simulink model "BE_EGAL_02"  (R2024b)
settings: Solver=ode45  StartTime=0.0  StopTime=Tfinal  RelTol=1e-3  EnableMultiTasking=on
values from neighbouring files (symbols this model uses):
  Constellation = exp(1i*pi*(1+2*kc)/4)    [init_ISI.m]
undefined symbols (not defined in the file or in its folder): dfilt, Limite, Tfinal
libraries: dspobslib x2, commdigbbndam3 x2, commchan3 x1, commsink2 x1, dspstat3 x1, commrandsrc3 x1
settings Model: Creator=Epsilon_2  LastModifiedBy=paulj
settings SolverCC: AlgebraicLoopSolver=TrustRegion
settings DataIOCC: LimitDataPoints=on  SaveFormat=Array  SignalLoggingSaveFormat=ModelDataLogs  SaveOutput=off  SaveTime=off  ReturnWorkspaceOutputs=off  SignalLoggingName=sigsOut
settings OptimizationCC: ExpressionDepthLimit=2147483647  InitFltsAndDblsToZero=on  LifeSpan=inf
settings DebuggingCC: SaveWithParameterizedLinksMsg=none  UnderspecifiedInitializationDetection=Classic  MergeDetectMultiDrivingBlocksExec=none  SignalResolutionControl=TryResolveAllWithWarning  MultiTaskDSMMsg=warning  MultiTaskCondExecSysMsg=none  FcnCallInpInsideContextMsg=warning  UnconnectedInputMsg=warning  UnconnectedOutputMsg=warning  UnconnectedLineMsg=warning  StateNameClashWarn=warning  SFUnexpectedBacktrackingDiag=warning  SFNoUnconditionalDefaultTransitionDiag=warning  ArithmeticOperatorsInVariantConditions=warning
settings HardwareCC: ProdBitPerPointer=32  ProdBitPerSizeT=32  ProdBitPerPtrDiffT=32  ProdLargestAtomicFloat=None  ProdIntDivRoundTo=Undefined  ProdEndianess=Unspecified  ProdWordSize=32  ProdHWDeviceType=32-bit Generic  TargetUnknown=on
settings ModelReferenceCC: EnableRefExpFcnMdlSchedulingChecks=on  PropagateSignalLabelsOutOfModel=off
settings SFSimCC: SimUseLocalCustomCode=off  CustomCodeUndefinedFunction=UseInterfaceOnly
settings RTWCC: RTWUseLocalCustomCode=off  GPUComputeCapability=3.5
settings CodeAppCC: StateflowObjectComments=on
settings GRTTargetCC: TargetFcnLib=ansi_tfl_tmw.mat  TargetLangStandard=C89/C90 (ANSI)  ModelReferenceCompliant=off  CombineOutputUpdateFcns=off  MatFileLogging=off  GRTInterface=on
settings ConfigComp: CovMetricSettings=dw  CovSaveCumulativeToWorkspaceVar=on  CovSaveSingleToWorkspaceVar=on  CovExternalEMLEnable=off

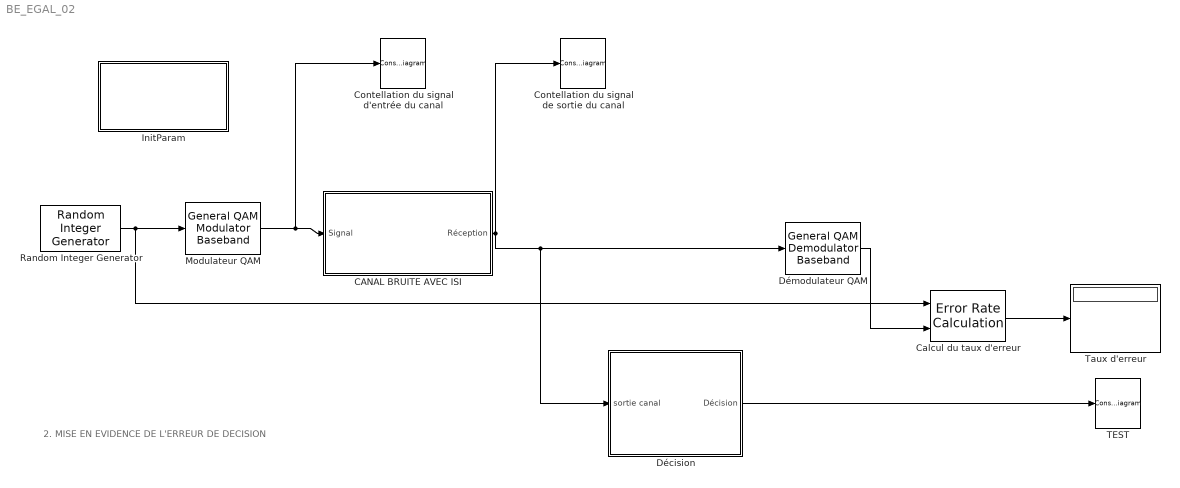
== system BE_EGAL_02 ==
  note: 2. MISE EN EVIDENCE DE L'ERREUR DE DECISION
  CANAL BRUITE AVEC ISI : Subsystem
  Calcul du taux d'erreur : commsink2/Error Rate Calculation  N=0  st_delay=0  cp_mode=Entire frame  subframe=[]  PMode=Port  WsName=ErrorVec  RsMode2=off  stop=off  numErr=100  maxBits=1e6
  Contellation du signal d'entrée du canal : ConstellationDiagram  Tag=ScatterPlot  WindowPosition=[232 118 560 560]  SymbolsToDisplaySource=Property  SymbolsToDisplay=Tfinal  Title=Constellation  XLimits=[-Limite Limite]  YLimits=[-Limite Limite]  ShowReferenceConstellation=off  DefaultConfigurationName=comm.scopes.ConstellationDiagramBlockCfg
  Contellation du signal de sortie du canal : ConstellationDiagram  Tag=ScatterPlot  WindowPosition=[232 118 560 560]  SymbolsToDisplaySource=Property  SymbolsToDisplay=Tfinal  Title=Constellation  XLimits=[-Limite Limite]  YLimits=[-Limite Limite]  ShowReferenceConstellation=off  DefaultConfigurationName=comm.scopes.ConstellationDiagramBlockCfg
  Décision : Subsystem
  "Démodulateur QAM " : commdigbbndam3/General QAM Demodulator Baseband  SigCon=Constellation  OutType=Integer  DecType=Hard decision  VarSource=Dialog  Variance=1  outDtypeBit=Inherit via internal rule  outDtype=double  roundingMode=Floor  overflowMode=Wrap  OvFlMode=off  OvFlModeLastStrValue=off  sigConstWordLen=16  sigConstDataTypeStr=Inherit: Same word length as input  sigConstLastDataTypeStr=Inherit: Same word length as input  accum1WordLen=32  accum1FracLen=30  prodInWordLen=32  prodInFracLen=30  prodInDataTypeStr=Inherit: Same as accumulator 1  prodInLastDataTypeStr=Inherit: Same as accumulator 1  prodOutWordLen=32  prodOutFracLen=30  accum2WordLen=32  accum2FracLen=30  accum3WordLen=32  accum3FracLen=30  nsiWordLen=32  nsiFracLen=30  nsiDataTypeStr=Inherit: Same as accumulator 3  nsiLastDataTypeStr=Inherit: Same as accumulator 3  invn0WordLen=16  invn0FracLen=8  invn0DataTypeStr=Inherit: Same word length as input  invn0LastDataTypeStr=Inherit: Same word length as input  outputWordLen=32  outputFracLen=30
  InitParam : Subsystem  mask{Tech=1, Tfinal=Tfinal, Mconst=4, NumCanal=[1 0.75 0.56 0.42 0.32 0.24 0.18], SNRcanal=0, NCoeffs=7, Kegal=0.02}
      mask prompts: Tech "Période de symbole"; Tfinal "Temps de simulation"; Mconst "Taille de la constellation de la modulation QAM : M (2^k)"; NumCanal "Modele RIF du canal"; SNRcanal "SNR du canal (en dB)"; NCoeffs "Nb de coefficients de l'égalisateur"; Kegal "Gain de l'égalisateur"
      mask help: Use the following mask to select the different parameters for the simulation.
      mask init:
      | eStr = init_ISI(gcb);
      mask Display: disp('Initialisation')
  "Modulateur QAM " : commdigbbndam3/General QAM Modulator Baseband  SigCon=Constellation  outDtype=double  outWordLen=16  outUDDataType=sfix(16)  outFracLenMode=Best precision  outFracLen=15  outDataTypeStr=double  outLastDataTypeStr=double
  Random Integer Generator : commrandsrc3/Random Integer Generator  SetSize=4  SeedSource=Auto  Seed=0  SampleTime=1  SamplesPerFrame=1  OutputDataType=double  SimulateUsing=Interpreted execution
  TEST : ConstellationDiagram  Tag=ScatterPlot  WindowPosition=[736.2 79.4 560 560]  SymbolsToDisplaySource=Property  SymbolsToDisplay=40  Title=Décision  XLimits=[-Limite Limite]  YLimits=[-Limite Limite]  ShowReferenceConstellation=off  ColorFading=on  DefaultConfigurationName=comm.scopes.ConstellationDiagramBlockCfg
  Taux d'erreur : Display
  wires:
  CANAL BRUITE AVEC ISI/1(Réception) -> Contellation du signal de sortie du canal/1, Décision/1(sortie canal), "Démodulateur QAM "/1
  Random Integer Generator/1 -> "Modulateur QAM "/1, Calcul du taux d'erreur/1
  "Modulateur QAM "/1 -> CANAL BRUITE AVEC ISI/1(Signal), Contellation du signal d'entrée du canal/1
  Calcul du taux d'erreur/1 -> Taux d'erreur/1
  "Démodulateur QAM "/1 -> Calcul du taux d'erreur/2
  Décision/1(Décision) -> TEST/1

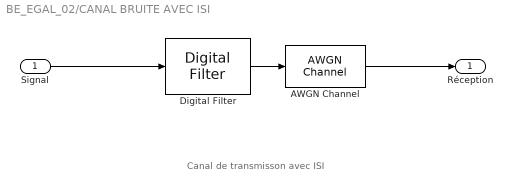
== system BE_EGAL_02/CANAL BRUITE AVEC ISI ==
  note: Canal de transmisson avec ISI
  Signal : Inport
  AWGN Channel : commchan3/AWGN Channel  InputProcessing=Inherited (this choice will be removed - see release notes)  seed=67  noiseMode="Signal to noise ratio  (SNR)"  EbNodB=10  EsNodB=10  SNRdB=SNRcanal  bitsPerSym=1  Ps=1  Tsym=1  variance=1
  Digital Filter : dspobslib/Digital Filter  TypePopup=FIR (all zeros)  IIRFiltStruct=Direct form II transposed  AllPoleFiltStruct=Direct form  FIRFiltStruct=Direct form  CoeffSource=Specify via dialog  NumCoeffs=NumCanal  DenCoeffs=[1 0.1]  BiQuadCoeffs=[1 0.3 0.4 1 0.1 0.2]  LatticeCoeffs=[0.2 0.4]  denIgnore=on  FiltPerSampPopup=One filter per sample  IC=0  ICnum=0  ICden=0  roundingMode=Floor  overflowMode=off  ScaleValues=1  scaleValueFracLength=14  stageInFracLength=15  stageOutFracLength=15  FilterSource=Specify via dialog  dfiltObjectName=dfilt.dffir([1 2 1])  InputProcessing=Inherited (this choice will be removed - see release notes)
  Réception : Outport
  wires:
  Digital Filter/1 -> AWGN Channel/1
  AWGN Channel/1 -> Réception/1
  Signal/1 -> Digital Filter/1

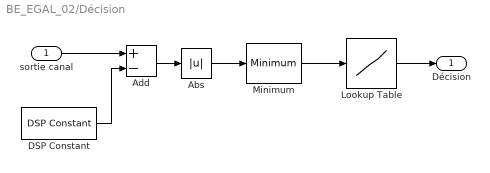
== system BE_EGAL_02/Décision ==
  sortie canal : Inport
  Abs : Abs  SaturateOnIntegerOverflow=off
  Add : Sum  Inputs=+-
  DSP Constant : dspobslib/DSP Constant  Value=Constellation  SampleMode=Discrete  discreteOutput=Sample-based (interpret vectors as 1-D)  continuousOutput=Sample-based  sampTime=inf  framePeriod=2  dataType=Inherit from 'Constant value'  isSigned=on  wordLen=16  udDataType=sfix(16)  fracBitsMode=Best precision  numFracBits=15  InterpretAs1D=-inf  Ts=-inf  FramebasedOutput=-inf
  Lookup Table : Lookup  InputValues=[1:4]  Table=Constellation  LookUpMeth=Use Input Nearest  SaturateOnIntegerOverflow=off
  Minimum : dspstat3/Minimum  fcn=Index  reset=None  InputProcessing=Columns as channels (frame based)  indexBase=One  operateOver=Each column  Dimension=1  operation=minimum  roiEnable=off  roiType=Rectangles  roiPortion=Entire ROI  roiOutput=Individual statistics for each ROI  roiFlag=off  roundingMode=Floor  overflowMode=off
  Décision : Outport
  wires:
  Minimum/1 -> Lookup Table/1
  Lookup Table/1 -> Décision/1
  Abs/1 -> Minimum/1
  Add/1 -> Abs/1
  DSP Constant/1 -> Add/2
  sortie canal/1 -> Add/1

== system BE_EGAL_02/InitParam ==
